simulink model "env"  (R2017a)
settings: Solver=FixedStepAuto  StartTime=0.0  StopTime=2  FixedStep=0.001  RelTol=1e-3
undefined symbols (not defined in the file): sigbuilder_block
libraries: simulink x1
settings Model: Creator=saturn  LastModifiedBy=saturn
settings DataIOCC: LimitDataPoints=on  SaveOutput=off  SaveTime=off
settings OptimizationCC: BlockReduction=off  BooleanDataType=off  LifeSpan=inf
settings DebuggingCC: SaveWithParameterizedLinksMsg=none  UnderspecifiedInitializationDetection=Classic  MergeDetectMultiDrivingBlocksExec=none  SignalResolutionControl=TryResolveAllWithWarning  AllowSymbolicDim=off  SFUnexpectedBacktrackingDiag=warning  SFNoUnconditionalDefaultTransitionDiag=warning  SFExecutionAtInitializationDiag=none
settings HardwareCC: TargetUnknown=on
settings GRTTargetCC: TargetLangStandard=C89/C90 (ANSI)  GeneratePreprocessorConditionals=Disable all

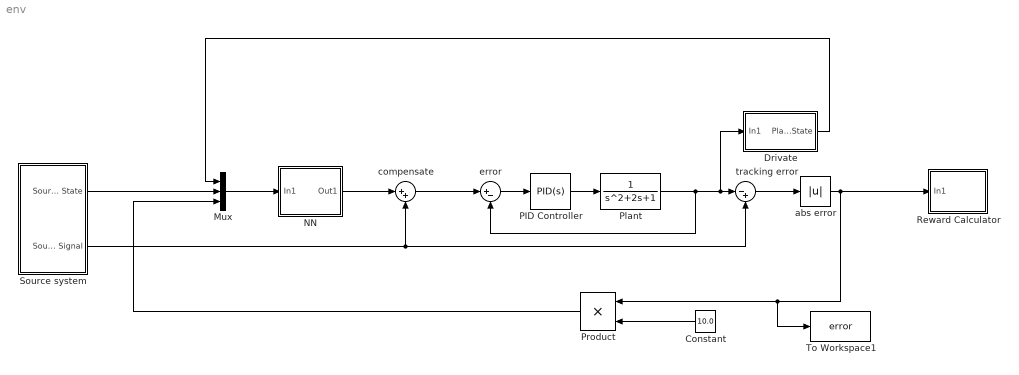
== system env ==
  Constant : Constant  Value=10.0
  "Drivate " : Subsystem
  Mux : Mux  Inputs=3
  NN : Subsystem
  PID Controller : simulink/Continuous/PID Controller  Controller=PID  TimeDomain=Continuous-time  SampleTime=-1  IntegratorMethod=Forward Euler  FilterMethod=Forward Euler  Form=Parallel  UseFilter=on  ControllerParametersSource=internal  P=2320.04721848328  I=12720.5381528177  D=103.291155860518  N=581.520102324439  InitialConditionSource=internal  InitialConditionForIntegrator=0  InitialConditionForFilter=0  ExternalReset=none  LimitOutput=off  UpperSaturationLimit=inf  LowerSaturationLimit=-inf  LinearizeAsGain=on  AntiWindupMode=none  Kb=1  TrackingMode=off  Kt=1  PParamMin=[]  PParamMax=[]  IParamMin=[]  IParamMax=[]  DParamMin=[]  DParamMax=[]  NParamMin=[]  NParamMax=[]  KbParamMin=[]  KbParamMax=[]  KtParamMin=[]  KtParamMax=[]  POutMin=[]  POutMax=[]  IOutMin=[]  IOutMax=[]  DOutMin=[]  DOutMax=[]  NOutMin=[]  NOutMax=[]  KbOutMin=[]  KbOutMax=[]  KtOutMin=[]  KtOutMax=[]  IntegratorOutMin=[]  IntegratorOutMax=[]  FilterOutMin=[]  FilterOutMax=[]  SumOutMin=[]  SumOutMax=[]  SumI1OutMin=[]  SumI1OutMax=[]  SumI2OutMin=[]  SumI2OutMax=[]  SumI3OutMin=[]  SumI3OutMax=[]  SumDOutMin=[]  SumDOutMax=[]  SaturationOutMin=[]  SaturationOutMax=[]  IntegratorContinuousStateAttributes=''  IntegratorStateMustResolveToSignalObject=off  IntegratorRTWStateStorageClass=Auto  FilterContinuousStateAttributes=''  FilterStateMustResolveToSignalObject=off  FilterRTWStateStorageClass=Auto  DifferentiatorICPrevScaledInput=0  DifferentiatorOutMin=[]  DifferentiatorOutMax=[]  InitialConditionSetting=State (most efficient)
  Plant : TransferFcn  Denominator=[ 1 2 1]  ContinuousStateAttributes='position'
  Product : Product
  "Reward Calculator " : Subsystem
  Source system : Subsystem
  To Workspace1 : ToWorkspace  VariableName=error  SaveFormat=Timeseries  SampleTime=-1
  abs error : Abs
  compensate : Sum  Inputs=|++
  error : Sum  Inputs=|+-
  tracking error : Sum  Inputs=|-+
  wires:
  Plant/1 -> error/2, "Drivate "/1(In1), tracking error/1
  error/1 -> PID Controller/1
  PID Controller/1 -> Plant/1
  Source system/2(Source Signal) -> compensate/2, tracking error/2
  compensate/1 -> error/1
  tracking error/1 -> abs error/1
  abs error/1 -> To Workspace1/1, Product/1, "Reward Calculator "/1(In1)
  "Drivate "/1(Plant State) -> Mux/1
  Source system/1("Source State ") -> Mux/2
  Constant/1 -> Product/2
  Product/1 -> Mux/3
  Mux/1 -> NN/1(In1)
  NN/1(Out1) -> compensate/1

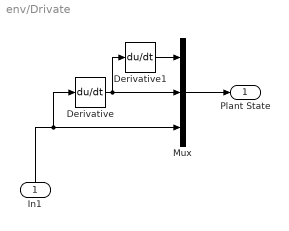
== system env/Drivate  ==
  In1 : Inport
  Derivative : Derivative
  Derivative1 : Derivative
  Mux : Mux  Inputs=3
  Plant State : Outport
  wires:
  Derivative1/1 -> Mux/1
  Mux/1 -> Plant State/1
  In1/1 -> Derivative/1, Mux/3
  Derivative/1 -> Derivative1/1, Mux/2

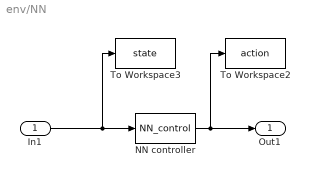
== system env/NN ==
  In1 : Inport
  NN controller : S-Function  FunctionName=NN_control  SFunctionDeploymentMode=off  EnableBusSupport=off
  To Workspace2 : ToWorkspace  VariableName=action  SaveFormat=Timeseries  SampleTime=-1
  To Workspace3 : ToWorkspace  VariableName=state  SaveFormat=Timeseries  SampleTime=-1
  Out1 : Outport
  wires:
  NN controller/1 -> Out1/1, To Workspace2/1
  In1/1 -> To Workspace3/1, NN controller/1

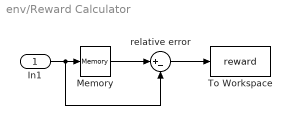
== system env/Reward Calculator  ==
  In1 : Inport
  Memory : Memory
  To Workspace : ToWorkspace  VariableName=reward  SaveFormat=Timeseries  SampleTime=-1
  "relative error " : Sum  Inputs=|+-
  wires:
  In1/1 -> Memory/1, "relative error "/2
  Memory/1 -> "relative error "/1
  "relative error "/1 -> To Workspace/1

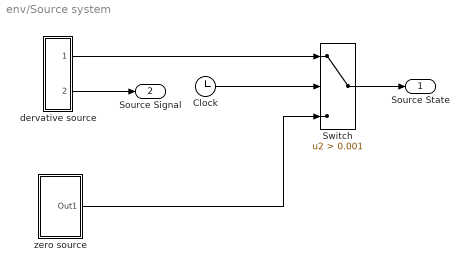
== system env/Source system ==
  Clock : Clock
  Switch : Switch  Criteria=u2 > Threshold  Threshold=0.001
  dervative source : Subsystem
  zero source : Subsystem
  "Source State " : Outport
  Source Signal : Outport  Port=2
  wires:
  Clock/1 -> Switch/2
  Switch/1 -> "Source State "/1
  dervative source/2(Out2) -> Source Signal/1
  zero source/1(Out1) -> Switch/3
  dervative source/1(Out1) -> Switch/1

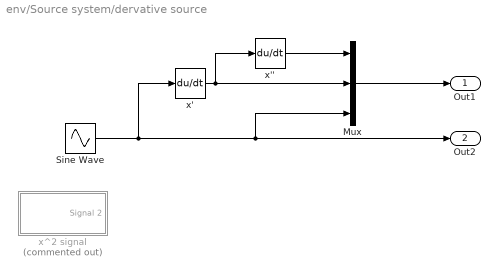
== system env/Source system/dervative source ==
  Mux : Mux  Inputs=3
  Sine Wave : Sin  Bias=-1  Frequency=pi/2  Phase=pi/2  SampleTime=0
  x' : Derivative
  x'' : Derivative
  x^2 signal : Subsystem  Tag=STV Subsys  Commented=on  LoadFcn=sigbuilder_block('load');  StartFcn=sigbuilder_block('start');  StopFcn=sigbuilder_block('stop');  ClipboardFcn=sigbuilder_block('clipboard');  mask(Sigbuilder block){tuvar=[0:10]}
      mask help: Simulink:masks:SigbuilderBlock_MD
      mask init:
      | if ~strcmp(get_param(bdroot(gcbh),'SimulationStatus'),'stopped') tuvar = sigbuilder_block('maskInit'); end
      settings: CopyFcn=sigbuilder_block('copy');  DeleteFcn=sigbuilder_block('delete');  ModelCloseFcn=sigbuilder_block('modelClose');  PreSaveFcn=sigbuilder_block('preSave');  PauseFcn=sigbuilder_block('pause');  ContinueFcn=sigbuilder_block('continue');  NameChangeFcn=sigbuilder_block('namechange');  OpenFcn=sigbuilder_block('open',[180.72 108.72 552.96 358.56 ]);  CloseFcn=sigbuilder_block('close');
      mask Display: plot(0, 0, 100, 100,[2, 2, 32, 32, 2], [68, 8, 8, 68, 68],[32, 2], [38, 38], [32, 19, 2],[53, 60, 44], [32, 17, 17, 2],[16, 16, 31, 31]);txt = getActiveGroup(gcbh);text(2, 100, txt,'verticalAlignment', 'top');
  Out1 : Outport
  Out2 : Outport  Port=2
  wires:
  Mux/1 -> Out1/1
  x'/1 -> Mux/2, x''/1
  x''/1 -> Mux/1
  Sine Wave/1 -> x'/1, Mux/3, Out2/1

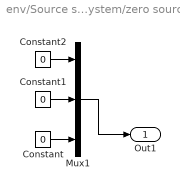
== system env/Source system/zero source ==
  Constant : Constant  Value=0
  Constant1 : Constant  Value=0
  Constant2 : Constant  Value=0
  Mux1 : Mux  Inputs=3
  Out1 : Outport
  wires:
  Constant1/1 -> Mux1/2
  Constant/1 -> Mux1/3
  Mux1/1 -> Out1/1
  Constant2/1 -> Mux1/1

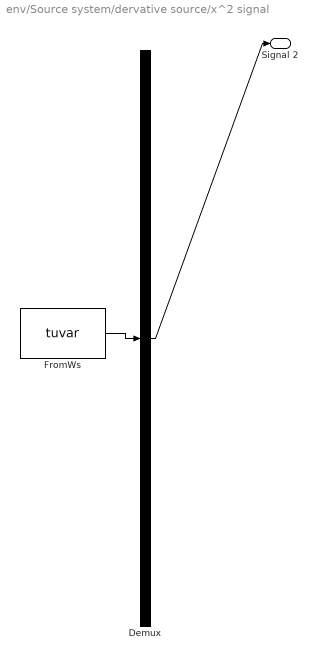
== system env/Source system/dervative source/x^2 signal ==
  Demux : Demux  Tag=STV Demux  Outputs=1
  FromWs : FromWorkspace  Tag=STV FromWs  VariableName=tuvar  SampleTime=0
      SigBuilderData=|
      | common.afterFinalStr = 'Extrapolate'
      | common.sampleTime = 0
      | dataSet.timeRange = [0 10]
      | dataSet.name = 'Group 1'
      | sbobj.Groups.Name = 'Group 1'
      | sbobj.Groups.Signals.Name = 'Signal 2'
      | sbobj.Groups.Signals.XData = [0 0.001 0.002 0.003 0.004 0.005 0.006 0.007 0.008 0.009 0.01 0.011 ... (10001 elements, 1x10001)]
      | sbobj.Groups.Signals.YData = [0 1e-06 4e-06 9e-06 1.6e-05 2.5e-05 3.6e-05 4.9e-05 6.4e-05 8.1e-05 0.0001 0.000121 ... (10001 elements, 1x10001)]
  Signal 2 : Outport  Tag=STV Outport
  wires:
  FromWs/1 -> Demux/1
  Demux/1 -> Signal 2/1
